simulink model "calc_c1_coefficients"  (R2020b)
settings: Solver=FixedStepDiscrete  StartTime=0.0  StopTime=stopTime  FixedStep=2.0833333333333333e-05  RelTol=1e-3
values from neighbouring files (symbols this model uses):
  C1initphase = C1initphase + atan(CF/(-rzero))-atan((CF-p_img)/(-p_real))-atan((CF+p_img)/(-p_real))    [modelparameters.m]
  CF = 2*pi*cf    (= 6283.18530718)    [modelparameters.m]
  ipb = 0.2343 * (2*pi) * cf - 1104    (= 368.150317472)    [modelparameters.m]
  ipw = 1.01 * cf * (2*pi) - 50    (= 6296.01716025)    [modelparameters.m]
  order_of_zero = half_order_pole    (= 5)    [modelparameters.m]
  phase_init = 0    [modelparameters.m]
  rpa = 10^(log10(cf)*0.9 + 0.55)+ 2000    [modelparameters.m]
  sigma0 = 1/taumax    (= 333.333333333)    [modelparameters.m]
settings Model: Creator=Ross  LastModifiedBy=conno
settings DataIOCC: SaveOutput=off  SaveTime=off  ReturnWorkspaceOutputs=off
settings OptimizationCC: BlockReduction=off  ConditionallyExecuteInputs=off  DefaultParameterBehavior=Inlined
settings DebuggingCC: ReadBeforeWriteMsg=DisableAll  WriteAfterWriteMsg=DisableAll  WriteAfterReadMsg=DisableAll  AlgebraicLoopMsg=error  MultiTaskDSMMsg=none  SingleTaskRateTransMsg=error  PregeneratedLibrarySubsystemCodeDiagnostic=none  ArithmeticOperatorsInVariantConditions=warning
settings HardwareCC: ProdBitPerPointer=32  ProdBitPerSizeT=32  ProdBitPerPtrDiffT=32  ProdLargestAtomicFloat=None  ProdIntDivRoundTo=Undefined  ProdEndianess=Unspecified  ProdWordSize=32  ProdHWDeviceType=ASIC/FPGA->ASIC/FPGA  TargetBitPerPointer=64  TargetBitPerSizeT=64  TargetBitPerPtrDiffT=64  TargetLongLongMode=on  TargetIntDivRoundTo=Zero  TargetEndianess=LittleEndian  TargetWordSize=64  TargetHWDeviceType=Custom Processor->MATLAB Host Computer  ProdEqTarget=off
settings ModelReferenceCC: UpdateModelReferenceTargets=IfOutOfDate  ModelReferenceNumInstancesAllowed=Single
settings SFSimCC: SFSimEcho=off  SimUseLocalCustomCode=off  CustomCodeUndefinedFunction=UseInterfaceOnly
settings RTWCC: RTWUseLocalCustomCode=off

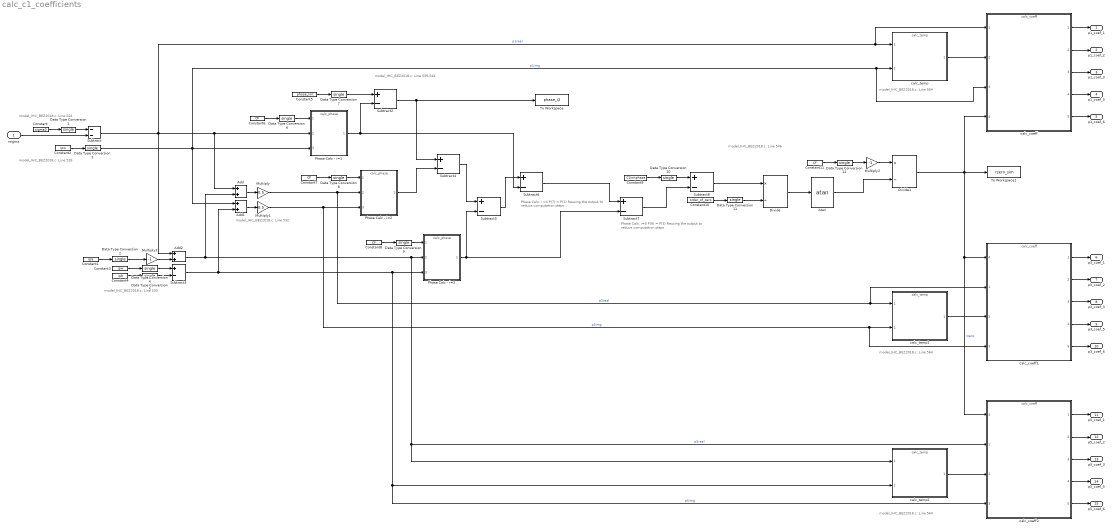
== system calc_c1_coefficients ==
  note: Phase Calc: i =4
      | P(7) = P(1)
      | Reusing the output to reduce computation steps
  note: model_IHC_BEZ2018.c: Line 524
  note: model_IHC_BEZ2018.c: Line 530
  note: model_IHC_BEZ2018.c: Line 532
  note: model_IHC_BEZ2018.c: Line 528
  note: Phase Calc: i=5
      | P(9) = P(5)
      | Reusing the output to reduce computation steps
  note: model_IHC_BEZ2018.c: Line 539-544
  note: model_IHC_BEZ2018.c: Line 546
  note: model_IHC_BEZ2018.c: Line 564
  note: model_IHC_BEZ2018.c: Line 564
  note: model_IHC_BEZ2018.c: Line 564
  rsigma : Inport  OutDataTypeStr=single  PortDimensions=1  SampleTime=[2.0833333333333333e-05,0]
  Add : Sum
  Add1 : Sum
  Add2 : Sum
  Atan : Trigonometry  Operator=atan
  Constant : Constant  Value=sigma0  SampleTime=-1
  Constant1 : Constant  Value=rpa  SampleTime=-1
  Constant10 : Constant  Value=order_of_zero  SampleTime=-1
  Constant{6..8,11} (4 alike) : Constant  Value=CF  SampleTime=-1
  Constant2 : Constant  Value=ipw  SampleTime=-1
  Constant3 : Constant  Value=ipw  SampleTime=-1
  Constant4 : Constant  Value=ipb  SampleTime=-1
  Constant5 : Constant  Value=phase_init  SampleTime=-1
  Constant9 : Constant  Value=C1initphase  SampleTime=-1
  Data Type Conversion{1..12} (12 alike) : DataTypeConversion  OutDataTypeStr=single  RndMeth=Nearest
  Divide : Product  Inputs=*/
  Divide1 : Product  Inputs=*/
  Multiply : Gain  Gain=0.5  OutDataTypeStr=Inherit: Same as input
  Multiply1 : Gain  Gain=0.5  OutDataTypeStr=Inherit: Same as input
  Multiply2 : Gain  Gain=-1
  Multiply3 : Gain  Gain=-1
  Phase Calc - i=1 : ModelReference  ModelNameDialog=calc_phase  SimulationMode=Normal  ModelReferenceVersion=1.134
  Phase Calc - i=2 : ModelReference  ModelNameDialog=calc_phase  SimulationMode=Normal  ModelReferenceVersion=1.134
  Phase Calc - i=3 : ModelReference  ModelNameDialog=calc_phase  SimulationMode=Normal  ModelReferenceVersion=1.134
  Subtract : Sum  Inputs=--
  Subtract{2..8} (7 alike) : Sum  Inputs=+-
  To Workspace : ToWorkspace  VariableName=phase_i2  SampleTime=-1
  To Workspace1 : ToWorkspace  VariableName=rzero_sim  SampleTime=-1
  calc_coeff : ModelReference  ModelNameDialog=calc_coeff  SimulationMode=Normal  ModelReferenceVersion=1.134
  calc_coeff1 : ModelReference  ModelNameDialog=calc_coeff  SimulationMode=Normal  ModelReferenceVersion=1.134
      settings: PortSchema="{\"entries\":[{\"content\":{\"sides\":[{\"content\":{\"connectorIds\":[\"In4\",\"In1\",\"In2\",\"In3\"]},\"type\":\"ConnectorPlacement.EquallySpacedRectSide\",\"uuid\":\"4b484a09-a038-445f-a06a-2e7f321aa8ef\"},{\"content\":{\"connectorIds\":[\"Out1\",\"Out2\",\"Out3\",\"Out4\",\"Out5\"],\"side\":\"RIGHT\"},\"type\":\"ConnectorPlacement.EquallySpacedRectSide\",\"uuid\":\"267f4d32-c4ed-453c-a2a5-fc1f2aa51a5b\"},{\"content\":{\"connectorIds\":[],\"side\":\"TOP\"},\"type\":\"ConnectorPlacement.EquallySpacedRectSide\",\"uuid\":\"f6362dc5-fbc9-40db-9e36-7c8e980642e3\"},{\"content\":{\"connectorIds\":[],\"side\":\"HIDDEN\"},\"type\":\"ConnectorPlacement.EquallySpacedRectSide\",\"uuid\":\"e088964f-f2f9-4d15-959e-ccd08d6e4837\"}]},\"type\":\"ConnectorPlacement.EquallySpacedConnector\",\"uuid\":\"d5aefeee-7e1a-4d9a-acb3-20dccb4230b6\"}],\"packageUris\":[\"http://schema.mathworks.com/mf0/Connector/R2020b\"],\"version\":\"1.0\"}"
  calc_coeff2 : ModelReference  ModelNameDialog=calc_coeff  SimulationMode=Normal  ModelReferenceVersion=1.134
      settings: PortSchema="{\"entries\":[{\"content\":{\"sides\":[{\"content\":{\"connectorIds\":[\"In4\",\"In1\",\"In2\",\"In3\"]},\"type\":\"ConnectorPlacement.EquallySpacedRectSide\",\"uuid\":\"4b484a09-a038-445f-a06a-2e7f321aa8ef\"},{\"content\":{\"connectorIds\":[\"Out1\",\"Out2\",\"Out3\",\"Out4\",\"Out5\"],\"side\":\"RIGHT\"},\"type\":\"ConnectorPlacement.EquallySpacedRectSide\",\"uuid\":\"267f4d32-c4ed-453c-a2a5-fc1f2aa51a5b\"},{\"content\":{\"connectorIds\":[],\"side\":\"TOP\"},\"type\":\"ConnectorPlacement.EquallySpacedRectSide\",\"uuid\":\"f6362dc5-fbc9-40db-9e36-7c8e980642e3\"},{\"content\":{\"connectorIds\":[],\"side\":\"HIDDEN\"},\"type\":\"ConnectorPlacement.EquallySpacedRectSide\",\"uuid\":\"e088964f-f2f9-4d15-959e-ccd08d6e4837\"}]},\"type\":\"ConnectorPlacement.EquallySpacedConnector\",\"uuid\":\"d5aefeee-7e1a-4d9a-acb3-20dccb4230b6\"}],\"packageUris\":[\"http://schema.mathworks.com/mf0/Connector/R2020b\"],\"version\":\"1.0\"}"
  calc_temp : ModelReference  ModelNameDialog=calc_temp  SimulationMode=Normal  ModelReferenceVersion=1.134
  calc_temp1 : ModelReference  ModelNameDialog=calc_temp  SimulationMode=Normal  ModelReferenceVersion=1.134
  calc_temp2 : ModelReference  ModelNameDialog=calc_temp  SimulationMode=Normal  ModelReferenceVersion=1.134
  p1_coef_1 : Outport
  p1_coef_2 : Outport  Port=2
  p1_coef_3 : Outport  Port=3
  p1_coef_5 : Outport  Port=4
  p1_coef_6 : Outport  Port=5
  p3_coef_1 : Outport  Port=6
  p3_coef_2 : Outport  Port=7
  p3_coef_3 : Outport  Port=8
  p3_coef_5 : Outport  Port=9
  p3_coef_6 : Outport  Port=10
  p5_coef_1 : Outport  Port=11
  p5_coef_2 : Outport  Port=12
  p5_coef_3 : Outport  Port=13
  p5_coef_5 : Outport  Port=14
  p5_coef_6 : Outport  Port=15
  wires:
  Data Type Conversion1/1 -> Subtract/1
  Subtract/1 -> Add2/1, calc_coeff/1, calc_temp/1, Add/1, Phase Calc - i=1/2  "p1real"
  Add/1 -> Multiply/1
  rsigma/1 -> Subtract/2
  Constant/1 -> Data Type Conversion1/1
  Data Type Conversion2/1 -> Multiply3/1
  Data Type Conversion3/1 -> calc_coeff/3, calc_temp/2, Add1/1, Phase Calc - i=1/3  "p1img"
  Constant2/1 -> Data Type Conversion3/1
  Constant3/1 -> Data Type Conversion4/1
  Data Type Conversion4/1 -> Subtract3/1
  Data Type Conversion5/1 -> Subtract3/2
  Constant4/1 -> Data Type Conversion5/1
  Multiply/1 -> Phase Calc - i=2/2, calc_temp1/1, calc_coeff1/1  "p3real"
  Add1/1 -> Multiply1/1
  Constant6/1 -> Data Type Conversion6/1
  Data Type Conversion6/1 -> Phase Calc - i=1/1
  Constant5/1 -> Data Type Conversion7/1
  Data Type Conversion7/1 -> Subtract2/1
  Phase Calc - i=1/1 -> Subtract6/2, Subtract2/2
  Subtract2/1 -> To Workspace/1, Subtract4/1
  Phase Calc - i=2/1 -> Subtract4/2
  Constant7/1 -> Data Type Conversion8/1
  Data Type Conversion8/1 -> Phase Calc - i=2/1
  Multiply1/1 -> Phase Calc - i=2/3, calc_temp1/2, calc_coeff1/3  "p3img"
  Data Type Conversion9/1 -> Phase Calc - i=3/1
  Constant8/1 -> Data Type Conversion9/1
  Subtract3/1 -> Add1/2, Phase Calc - i=3/3, calc_temp2/2, calc_coeff2/3  "p5img"
  Add2/1 -> Add/2, Phase Calc - i=3/2, calc_temp2/1, calc_coeff2/1  "p5real"
  Phase Calc - i=3/1 -> Subtract7/2, Subtract5/2
  Subtract4/1 -> Subtract5/1
  Subtract5/1 -> Subtract6/1
  Subtract6/1 -> Subtract7/1
  Constant9/1 -> Data Type Conversion10/1
  Data Type Conversion10/1 -> Subtract8/1
  Subtract7/1 -> Subtract8/2
  Subtract8/1 -> Divide/1
  Constant10/1 -> Data Type Conversion11/1
  Data Type Conversion11/1 -> Divide/2
  Divide/1 -> Atan/1
  Data Type Conversion12/1 -> Multiply2/1
  Constant11/1 -> Data Type Conversion12/1
  Multiply2/1 -> Divide1/1
  Atan/1 -> Divide1/2
  Divide1/1 -> To Workspace1/1, calc_coeff2/4, calc_coeff1/4, calc_coeff/4  "rzero"
  Constant1/1 -> Data Type Conversion2/1
  calc_temp/1 -> calc_coeff/2
  calc_coeff/1 -> p1_coef_1/1
  calc_coeff/2 -> p1_coef_2/1
  calc_coeff/3 -> p1_coef_3/1
  calc_coeff/4 -> p1_coef_5/1
  calc_coeff/5 -> p1_coef_6/1
  calc_coeff1/3 -> p3_coef_3/1
  calc_coeff1/5 -> p3_coef_6/1
  calc_coeff1/2 -> p3_coef_2/1
  calc_coeff1/1 -> p3_coef_1/1
  calc_temp1/1 -> calc_coeff1/2
  calc_coeff1/4 -> p3_coef_5/1
  calc_temp2/1 -> calc_coeff2/2
  calc_coeff2/4 -> p5_coef_5/1
  calc_coeff2/2 -> p5_coef_2/1
  calc_coeff2/1 -> p5_coef_1/1
  calc_coeff2/5 -> p5_coef_6/1
  calc_coeff2/3 -> p5_coef_3/1
  Multiply3/1 -> Add2/2
